simulink model "rlmodeltemplate"  (R2020a)
settings: Solver=VariableStepAuto  StartTime=0.0  StopTime=10.0  RelTol=1e-3
libraries: rllib x1
settings Model: Creator=The MathWorks, Inc.  LastModifiedBy=The MathWorks, Inc.
settings DataIOCC: ReturnWorkspaceOutputs=off
settings DebuggingCC: ArithmeticOperatorsInVariantConditions=warning
settings SFSimCC: CustomCodeUndefinedFunction=UseInterfaceOnly

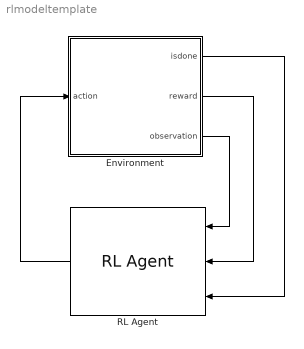
== system rlmodeltemplate ==
  Environment : Subsystem
  RL Agent : rllib/RL Agent  Agent=agent  ProvideReward=on  ProvideIsDone=on  ProvideCumRwd=off  TreatAsDirectFeedthrough=on  CollectLoggedSignals=on  CollectModelStates=on
  wires:
  Environment/3(observation) -> RL Agent/1
  Environment/2(reward) -> RL Agent/2
  Environment/1(isdone) -> RL Agent/3
  RL Agent/1 -> Environment/1(action)

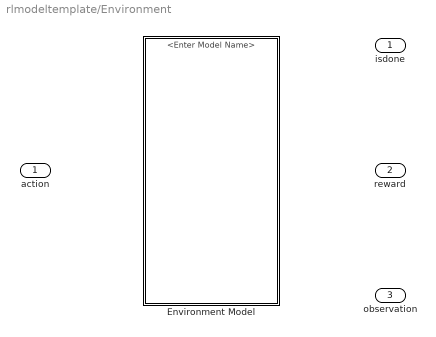
== system rlmodeltemplate/Environment ==
  action : Inport
  Environment Model : ModelReference  SimulationMode=Normal
  isdone : Outport  VectorParamsAs1DForOutWhenUnconnected=off
  reward : Outport  Port=2  VectorParamsAs1DForOutWhenUnconnected=off
  observation : Outport  Port=3  VectorParamsAs1DForOutWhenUnconnected=off
